simulink model "MRAC_Full_State"  (R2016b)
settings: Solver=ode23tb  StartTime=0.0  StopTime=50  RelTol=1e-3
undefined symbols (not defined in the file or in its folder): sigbuilder_block
settings Model: Creator=Niels  LastModifiedBy=Niels
settings SolverCC: ZeroCrossAlgorithm=Adaptive

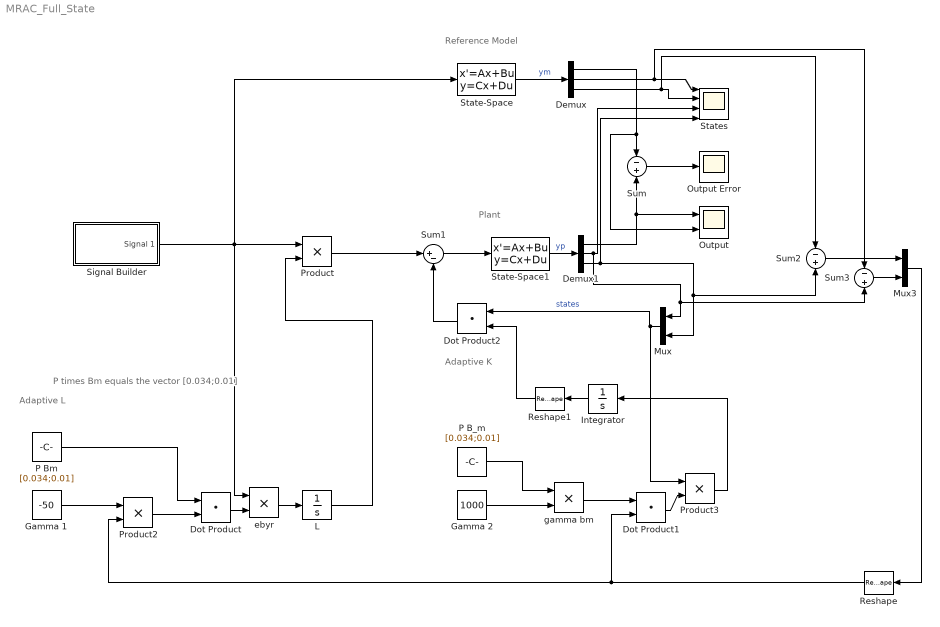
== system MRAC_Full_State ==
  note: Reference Model
  note: Plant
  note: Adaptive K
  note: P times Bm equals the vector [0.034;0.01]
  note: Adaptive L
  Demux : Demux  Outputs=3
  Demux1 : Demux  Outputs=3
  Dot Product : DotProduct  InputSameDT=on  OutDataTypeStr=Inherit: Inherit via internal rule
  Dot Product1 : DotProduct  InputSameDT=on  OutDataTypeStr=Inherit: Inherit via internal rule
  Dot Product2 : DotProduct  InputSameDT=on  OutDataTypeStr=Inherit: Inherit via internal rule
  Gamma 1 : Constant  Value=-50
  Gamma 2 : Constant  Value=1000
  Integrator : Integrator
  L : Integrator
  Mux : Mux  Inputs=2
  Mux3 : Mux  Inputs=2
  Output : Scope  NumInputPorts=2
  Output Error : Scope
  P B_m : Constant  Value=[0.034;0.01]
  P Bm : Constant  Value=[0.034;0.01]  VectorParams1D=off
  Product : Product
  Product2 : Product
  Product3 : Product
  Reshape : Reshape  OutputDimensionality=Row vector (2-D)  OutputDimensions=2
  Reshape1 : Reshape  OutputDimensionality=Row vector (2-D)
  Signal Builder : Subsystem  Tag=STV Subsys  LoadFcn=sigbuilder_block('load',[437.6 199.2 550.4 400 ]);  StartFcn=sigbuilder_block('start');  StopFcn=sigbuilder_block('stop');  ClipboardFcn=sigbuilder_block('clipboard');  mask(Sigbuilder block){tuvar=[0:10]}
      mask help: Simulink:masks:SigbuilderBlock_MD
      mask init:
      | if ~strcmp(get_param(bdroot(gcbh),'SimulationStatus'),'stopped') tuvar = sigbuilder_block('maskInit'); end
      settings: CopyFcn=sigbuilder_block('copy');  DeleteFcn=sigbuilder_block('delete');  ModelCloseFcn=sigbuilder_block('modelClose');  PreSaveFcn=sigbuilder_block('preSave');  PauseFcn=sigbuilder_block('pause');  ContinueFcn=sigbuilder_block('continue');  NameChangeFcn=sigbuilder_block('namechange');  OpenFcn=sigbuilder_block('open',[437.6 199.2 550.4 400 ]);  CloseFcn=sigbuilder_block('close');
      mask Display: plot(0, 0, 100, 100,[2, 2, 32, 32, 2], [68, 8, 8, 68, 68],[32, 2], [38, 38], [32, 19, 2],[53, 60, 44], [32, 17, 17, 2],[16, 16, 31, 31]);txt = getActiveGroup(gcbh);text(2, 100, txt,'verticalAlignment', 'top');
  State-Space : StateSpace  A=[-15 -50;1 0]  B=[1;0]  C=[1 50;1 0;0 1]  D=[0;0;0]  X0=0
  State-Space1 : StateSpace  A=[-0.75 -2.5;1 0]  B=[1;0]  C=[1 1.5;1 0;0 1]  D=[0;0;0]  X0=[0.1;-0.1]
  States : Scope  NumInputPorts=4
  Sum : Sum  Inputs=-|+
  Sum1 : Sum  Inputs=|+-
  Sum2 : Sum  Inputs=-|+
  Sum3 : Sum  Inputs=-|+
  ebyr : Product
  gamma bm : Product
  wires:
  Sum/1 -> Output Error/1
  Sum1/1 -> State-Space1/1
  State-Space/1 -> Demux/1  "ym"
  Demux/1 -> Output/2, Sum/1
  Demux/2 -> Sum3/1, States/1
  Demux/3 -> Sum2/1, States/2
  State-Space1/1 -> Demux1/1  "yp"
  Demux1/2 -> Sum3/2, Mux/1, States/3
  Demux1/3 -> Sum2/2, Mux/2, States/4
  Demux1/1 -> Output/1, Sum/2
  Signal Builder/1(Signal 1) -> Product/1, ebyr/1, State-Space/1
  Product/1 -> Sum1/1
  Gamma 1/1 -> Product2/1
  Product2/1 -> Dot Product/2
  P Bm/1 -> Dot Product/1
  Dot Product/1 -> ebyr/2
  ebyr/1 -> L/1
  L/1 -> Product/2
  Gamma 2/1 -> gamma bm/2
  P B_m/1 -> gamma bm/1
  gamma bm/1 -> Dot Product1/1
  Dot Product1/1 -> Product3/2
  Mux/1 -> Product3/1, Dot Product2/1  "states"
  Product3/1 -> Integrator/1
  Dot Product2/1 -> Sum1/2
  Sum3/1 -> Mux3/2
  Sum2/1 -> Mux3/1
  Mux3/1 -> Reshape/1
  Reshape/1 -> Dot Product1/2, Product2/2
  Integrator/1 -> Reshape1/1
  Reshape1/1 -> Dot Product2/2

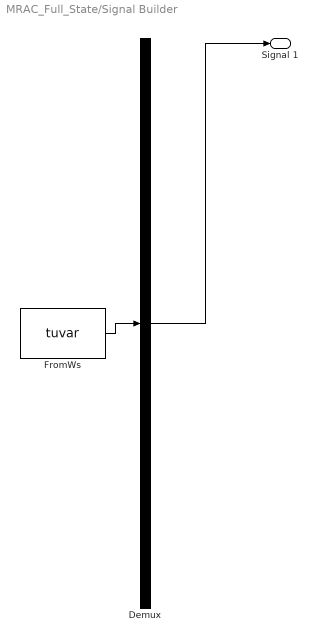
== system MRAC_Full_State/Signal Builder ==
  Demux : Demux  Tag=STV Demux  Outputs=1
  FromWs : FromWorkspace  Tag=STV FromWs  VariableName=tuvar  SampleTime=0
      SigBuilderData=|
      | common.afterFinalStr = 'Extrapolate'
      | common.sampleTime = 0
      | dataSet.timeRange = [0 10]
      | dataSet.name = 'Group 1'
      | sbobj.Groups.Name = 'Group 1'
      | sbobj.Groups.Signals.Name = 'Signal 1'
      | sbobj.Groups.Signals.XData = [0 0.88 0.88 10]
      | sbobj.Groups.Signals.YData = [0 0 10 10]
  Signal 1 : Outport  Tag=STV Outport
  wires:
  Demux/1 -> Signal 1/1
  FromWs/1 -> Demux/1
